simulink model "mavsim_manual_multi"  (R2016b)
settings: Solver=ode15s  StartTime=0.0  StopTime=10000  RelTol=1e-3  EnableMultiTasking=on
InitFcn:
  | param
values from neighbouring files (symbols this model uses):
  P = GenCoefs(P)    [param.m]    (also in param_chap5.m)
undefined symbols (not defined in the file or in its folder): autopilot, drawAircraft, estimate_states, forces_moments, gps, plane_follow, plotextramavstatevariables, plotmavstatevariables, sensors, true_states
libraries: simulink x9
settings Model: Creator=beard  LastModifiedBy=Brian Jackson
settings DataIOCC: LimitDataPoints=on  SaveFormat=Array  SignalLoggingSaveFormat=ModelDataLogs
settings OptimizationCC: ExpressionDepthLimit=2147483647  InitFltsAndDblsToZero=on  LifeSpan=inf
settings DebuggingCC: UnderspecifiedInitializationDetection=Classic  MergeDetectMultiDrivingBlocksExec=none  SolverPrmCheckMsg=warning  FcnCallInpInsideContextMsg=warning  StateNameClashWarn=warning  SFUnexpectedBacktrackingDiag=warning  SFNoUnconditionalDefaultTransitionDiag=warning  SFExecutionAtInitializationDiag=none
settings HardwareCC: ProdBitPerPointer=32  ProdBitPerSizeT=32  ProdBitPerPtrDiffT=32  ProdLargestAtomicFloat=None  ProdIntDivRoundTo=Undefined  ProdEndianess=Unspecified  ProdWordSize=32  ProdHWDeviceType=32-bit Generic
settings ModelReferenceCC: PropagateSignalLabelsOutOfModel=off
settings GRTTargetCC: TargetLangStandard=C89/C90 (ANSI)  GeneratePreprocessorConditionals=Disable all  CombineOutputUpdateFcns=off  GRTInterface=on
settings ConfigComp: CovMetricSettings=dw  CovHtmlReporting=on  CovSaveCumulativeToWorkspaceVar=on  CovSaveSingleToWorkspaceVar=on  CovExternalEMLEnable=off  CovSFcnEnable=off

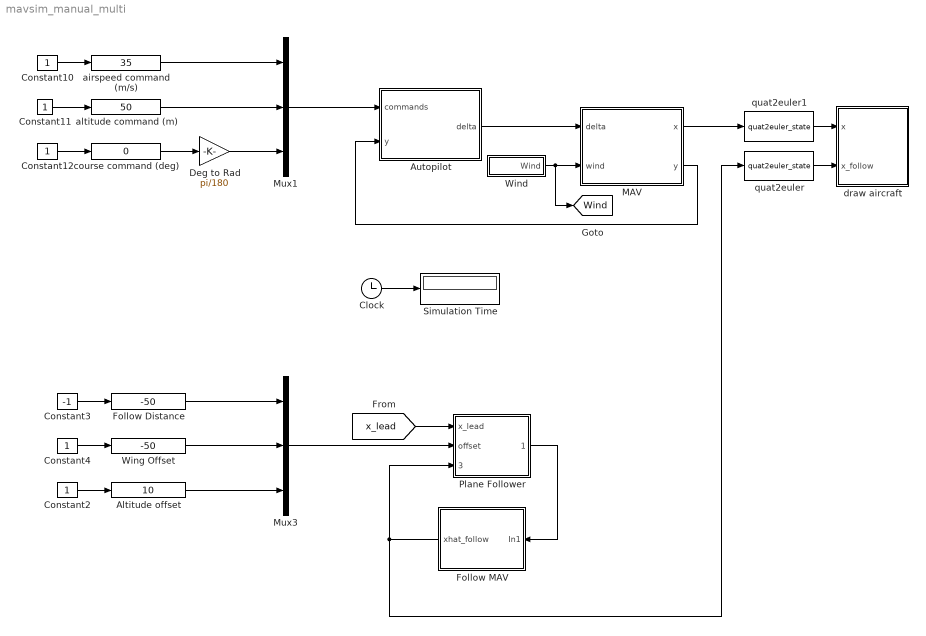
== system mavsim_manual_multi ==
  Altitude offset : simulink/Math Operations/Slider Gain  low=0  gain=10  high=10
  Autopilot : Subsystem
      mask Display: image(imread('kestrel.jpg'))
  Clock : Clock
  Constant{2,4,10..12} (5 alike) : Constant
  Constant3 : Constant  Value=-1
  Deg to Rad : Gain  Gain=pi/180
  Follow Distance : simulink/Math Operations/Slider Gain  low=-50  gain=-50  high=50
  Follow MAV : Subsystem
      mask Display: image(imread('batcam.png'))
  MAV : Subsystem
      mask Display: image(imread('batcam.png'))
  Mux1 : Mux  Inputs=3
  Mux3 : Mux  Inputs=3
  Plane Follower : Subsystem
  Simulation Time : Display
  Wind : Subsystem
  Wing Offset : simulink/Math Operations/Slider Gain  low=-50  gain=-50  high=50
  airspeed command (m/s) : simulink/Math Operations/Slider Gain  low=5  gain=35  high=50
  altitude command (m) : simulink/Math Operations/Slider Gain  low=-50  gain=50  high=500
  course command (deg) : simulink/Math Operations/Slider Gain  low=-360  gain=0  high=360
  draw aircraft : Subsystem
      mask Display: image(imread('tv.png'))
  quat2euler : MATLABFcn  MATLABFcn=quat2euler_state
  "quat2euler1 " : MATLABFcn  MATLABFcn=quat2euler_state
  tag scope: Wind=global
  wires:
  Clock/1 -> Simulation Time/1
  Autopilot/1(delta) -> MAV/1(delta)
  "quat2euler1 "/1 -> draw aircraft/1(x)
  Constant10/1 -> airspeed command (m/s)/1
  Constant11/1 -> altitude command (m)/1
  Constant12/1 -> course command (deg)/1
  course command (deg)/1 -> Deg to Rad/1
  altitude command (m)/1 -> Mux1/2
  airspeed command (m/s)/1 -> Mux1/1
  Deg to Rad/1 -> Mux1/3
  Mux1/1 -> Autopilot/1(commands)
  MAV/1(x) -> "quat2euler1 "/1
  MAV/2(y) -> Autopilot/2(y)
  Constant2/1 -> Altitude offset/1
  Constant3/1 -> Follow Distance/1
  Constant4/1 -> Wing Offset/1
  Follow Distance/1 -> Mux3/1
  Wing Offset/1 -> Mux3/2
  Altitude offset/1 -> Mux3/3
  quat2euler/1 -> draw aircraft/2(x_follow)
  Wind/1(Wind) -> [Wind], MAV/2(wind)
  [x_lead] -> Plane Follower/1(x_lead)
  Mux3/1 -> Plane Follower/2(offset)
  Follow MAV/1(xhat_follow) -> Plane Follower/3(x_follow), quat2euler/1
  Plane Follower/1(commands) -> Follow MAV/1(In1)

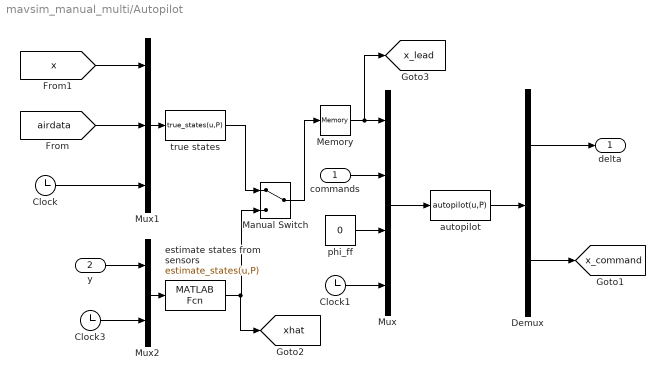
== system mavsim_manual_multi/Autopilot ==
  commands : Inport
  y : Inport  Port=2
  Clock : Clock
  Clock1 : Clock
  Clock3 : Clock
  Demux : Demux  Outputs=[4;12]
  Manual Switch : ManualSwitch
  Memory : Memory
  Mux : Mux
  Mux1 : Mux  Inputs=3
  Mux2 : Mux  Inputs=2
  autopilot : MATLABFcn  MATLABFcn=autopilot(u,P)  OutputDimensions=4+12  SampleTime=P.Ts
  estimate states from sensors : MATLABFcn  MATLABFcn=estimate_states(u,P)  OutputDimensions=19  SampleTime=P.Ts
  phi_ff : Constant  Value=0
  true states : MATLABFcn  MATLABFcn=true_states(u,P)  OutputDimensions=19  SampleTime=P.Ts
  delta : Outport
  tag scope: x_command=global, x_lead=global, xhat=global
  wires:
  Mux/1 -> autopilot/1
  Clock/1 -> Mux1/3
  autopilot/1 -> Demux/1
  Demux/1 -> delta/1
  Demux/2 -> [x_command]
  commands/1 -> Mux/2
  Mux1/1 -> true states/1
  [x] -> Mux1/1
  [airdata] -> Mux1/2
  Memory/1 -> [x_lead], Mux/1
  Clock1/1 -> Mux/4
  Mux2/1 -> estimate states from sensors/1
  y/1 -> Mux2/1
  Clock3/1 -> Mux2/2
  true states/1 -> Manual Switch/1
  estimate states from sensors/1 -> [xhat], Manual Switch/2
  Manual Switch/1 -> Memory/1
  phi_ff/1 -> Mux/3

== system mavsim_manual_multi/Follow MAV ==
  In1 : Inport
  Autopilot_follow : Subsystem
      mask Display: image(imread('kestrel.jpg'))
  MAV_follow : Subsystem
      mask Display: image(imread('batcam.png'))
  xhat_follow : Outport
  wires:
  In1/1 -> Autopilot_follow/1(commands)
  MAV_follow/1(y) -> Autopilot_follow/2(y)
  Autopilot_follow/2(delta) -> MAV_follow/1(delta)
  [Wind] -> MAV_follow/2(wind)
  Autopilot_follow/1(xhat_follow) -> xhat_follow/1

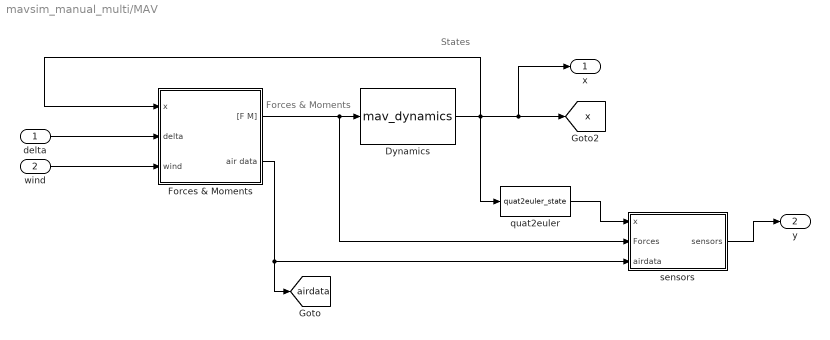
== system mavsim_manual_multi/MAV ==
  note: Forces & Moments
  note: States
  delta : Inport
  wind : Inport  Port=2
  Dynamics : S-Function  FunctionName=mav_dynamics  Parameters=P  SFunctionDeploymentMode=off  EnableBusSupport=off
  Forces & Moments : Subsystem
  "quat2euler " : MATLABFcn  MATLABFcn=quat2euler_state
  sensors : Subsystem
  x : Outport
  y : Outport  Port=2
  tag scope: airdata=global, x=global
  wires:
  Dynamics/1 -> x/1, [x], Forces & Moments/1(x), "quat2euler "/1
  Forces & Moments/1("[F M]") -> sensors/2(Forces), Dynamics/1
  Forces & Moments/2(air data) -> sensors/3(airdata), [airdata]
  delta/1 -> Forces & Moments/2(delta)
  wind/1 -> Forces & Moments/3(wind)
  "quat2euler "/1 -> sensors/1(x)
  sensors/1(sensors) -> y/1

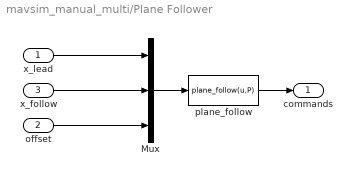
== system mavsim_manual_multi/Plane Follower ==
  x_lead : Inport
  offset : Inport  Port=2
  x_follow : Inport  Port=3
  Mux : Mux  Inputs=3
  plane_follow : MATLABFcn  MATLABFcn=plane_follow(u,P)  OutputDimensions=4
  commands : Outport
  wires:
  offset/1 -> Mux/3
  Mux/1 -> plane_follow/1
  x_lead/1 -> Mux/1
  x_follow/1 -> Mux/2
  plane_follow/1 -> commands/1

== system mavsim_manual_multi/Wind ==
  Constant1 : Constant  Value=[0; 0; 0]
  Constant2 : Constant  Value=[P.wind_n; P.wind_e; P.wind_d]
  Mux1 : Mux  Inputs=2
  Wind Gusts : Subsystem
  Wind : Outport
  wires:
  Constant2/1 -> Mux1/1
  Mux1/1 -> Wind/1
  Constant1/1 -> Mux1/2

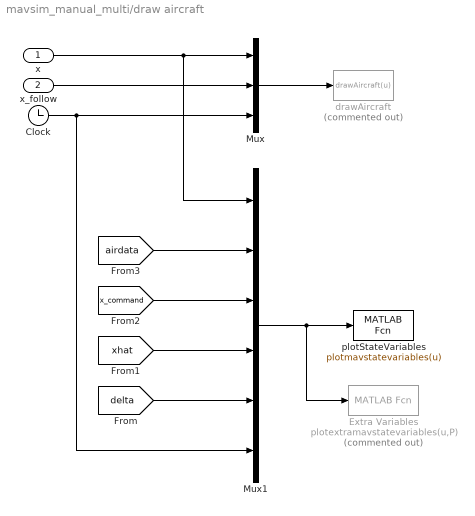
== system mavsim_manual_multi/draw aircraft ==
  x : Inport
  x_follow : Inport  Port=2
  Clock : Clock
  Extra Variables : MATLABFcn  Commented=on  MATLABFcn=plotextramavstatevariables(u,P)  OutputDimensions=0
  Mux : Mux  Inputs=3
  Mux1 : Mux  Inputs=6
  drawAircraft : MATLABFcn  Commented=on  MATLABFcn=drawAircraft(u)  OutputDimensions=0  SampleTime=0.1
  plotStateVariables : MATLABFcn  MATLABFcn=plotmavstatevariables(u)  OutputDimensions=0  SampleTime=0.1
  wires:
  Mux/1 -> drawAircraft/1
  x/1 -> Mux1/1, Mux/1
  Clock/1 -> Mux/3, Mux1/6
  Mux1/1 -> Extra Variables/1, plotStateVariables/1
  [xhat] -> Mux1/4
  [x_command] -> Mux1/3
  [delta] -> Mux1/5
  [airdata] -> Mux1/2
  x_follow/1 -> Mux/2

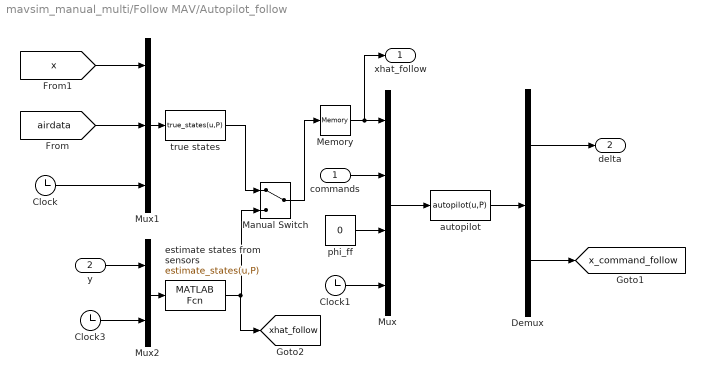
== system mavsim_manual_multi/Follow MAV/Autopilot_follow ==
  commands : Inport
  y : Inport  Port=2
  Clock : Clock
  Clock1 : Clock
  Clock3 : Clock
  Demux : Demux  Outputs=[4;12]
  Manual Switch : ManualSwitch
  Memory : Memory
  Mux : Mux
  Mux1 : Mux  Inputs=3
  Mux2 : Mux  Inputs=2
  autopilot : MATLABFcn  MATLABFcn=autopilot(u,P)  OutputDimensions=4+12  SampleTime=P.Ts
  estimate states from sensors : MATLABFcn  MATLABFcn=estimate_states(u,P)  OutputDimensions=19  SampleTime=P.Ts
  phi_ff : Constant  Value=0
  true states : MATLABFcn  MATLABFcn=true_states(u,P)  OutputDimensions=19  SampleTime=P.Ts
  xhat_follow : Outport
  delta : Outport  Port=2
  tag scope: x_command_follow=global, xhat_follow=global
  wires:
  Mux/1 -> autopilot/1
  Clock/1 -> Mux1/3
  autopilot/1 -> Demux/1
  Demux/1 -> delta/1
  Demux/2 -> [x_command_follow]
  commands/1 -> Mux/2
  Mux1/1 -> true states/1
  [x] -> Mux1/1
  [airdata] -> Mux1/2
  Memory/1 -> xhat_follow/1, Mux/1
  Clock1/1 -> Mux/4
  Mux2/1 -> estimate states from sensors/1
  y/1 -> Mux2/1
  Clock3/1 -> Mux2/2
  true states/1 -> Manual Switch/1
  estimate states from sensors/1 -> [xhat_follow], Manual Switch/2
  Manual Switch/1 -> Memory/1
  phi_ff/1 -> Mux/3

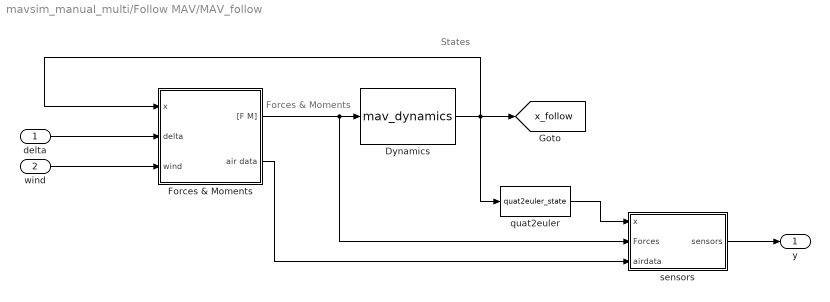
== system mavsim_manual_multi/Follow MAV/MAV_follow ==
  note: Forces & Moments
  note: States
  delta : Inport
  wind : Inport  Port=2
  Dynamics : S-Function  FunctionName=mav_dynamics  Parameters=P  SFunctionDeploymentMode=off  EnableBusSupport=off
  Forces & Moments : Subsystem
  "quat2euler " : MATLABFcn  MATLABFcn=quat2euler_state
  sensors : Subsystem
  y : Outport
  tag scope: x_follow=global
  wires:
  Dynamics/1 -> [x_follow], Forces & Moments/1(x), "quat2euler "/1
  Forces & Moments/1("[F M]") -> sensors/2(Forces), Dynamics/1
  Forces & Moments/2(air data) -> sensors/3(airdata)
  delta/1 -> Forces & Moments/2(delta)
  wind/1 -> Forces & Moments/3(wind)
  "quat2euler "/1 -> sensors/1(x)
  sensors/1(sensors) -> y/1

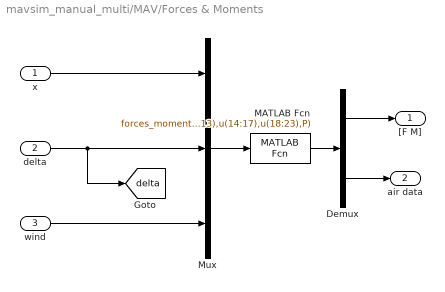
== system mavsim_manual_multi/MAV/Forces & Moments ==
  x : Inport
  delta : Inport  Port=2
  wind : Inport  Port=3
  Demux : Demux  Outputs=[6;6]
  MATLAB Fcn : MATLABFcn  MATLABFcn=forces_moments(u(1:13),u(14:17),u(18:23),P)  OutputDimensions=12
  Mux : Mux  Inputs=3
  "[F M]" : Outport
  air data : Outport  Port=2
  tag scope: delta=global
  wires:
  Demux/2 -> air data/1
  Mux/1 -> MATLAB Fcn/1
  Demux/1 -> "[F M]"/1
  MATLAB Fcn/1 -> Demux/1
  wind/1 -> Mux/3
  delta/1 -> Mux/2, [delta]
  x/1 -> Mux/1

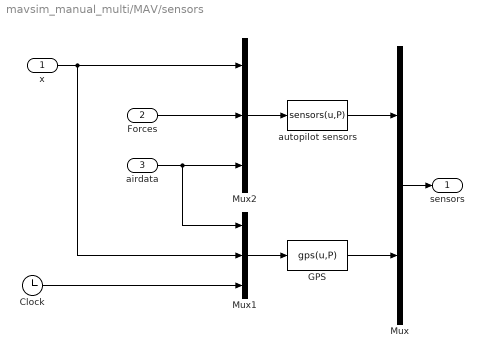
== system mavsim_manual_multi/MAV/sensors ==
  x : Inport
  Forces : Inport  Port=2
  airdata : Inport  Port=3
  Clock : Clock
  GPS : MATLABFcn  MATLABFcn=gps(u,P)  OutputDimensions=5  SampleTime=P.Ts_gps
  Mux : Mux  Inputs=2
  Mux1 : Mux  Inputs=3
  Mux2 : Mux  Inputs=3
  autopilot sensors : MATLABFcn  MATLABFcn=sensors(u,P)  OutputDimensions=8  SampleTime=P.Ts
  sensors : Outport
  wires:
  autopilot sensors/1 -> Mux/1
  GPS/1 -> Mux/2
  Mux1/1 -> GPS/1
  Clock/1 -> Mux1/3
  Mux2/1 -> autopilot sensors/1
  Forces/1 -> Mux2/2
  airdata/1 -> Mux2/3, Mux1/1
  Mux/1 -> sensors/1
  x/1 -> Mux2/1, Mux1/2

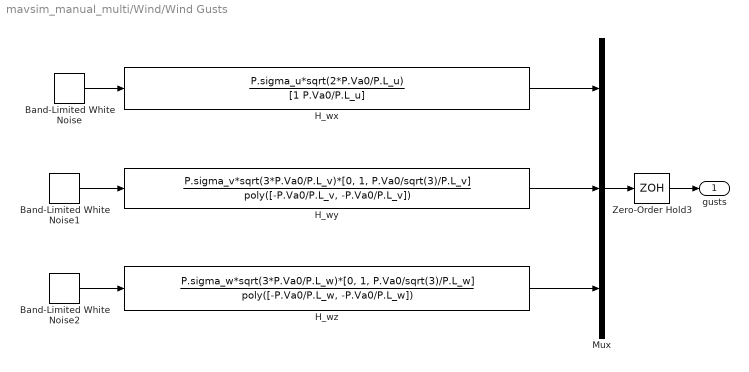
== system mavsim_manual_multi/Wind/Wind Gusts ==
  Band-Limited White Noise : simulink/Sources/Band-Limited White Noise  Cov=[1]  Ts=P.Ts  seed=[23341]
  Band-Limited White Noise1 : simulink/Sources/Band-Limited White Noise  Cov=[1]  Ts=P.Ts  seed=[23341]
  Band-Limited White Noise2 : simulink/Sources/Band-Limited White Noise  Cov=[1]  Ts=P.Ts  seed=[23341]
  H_wx : TransferFcn  Numerator=P.sigma_u*sqrt(2*P.Va0/P.L_u)  Denominator=[1 P.Va0/P.L_u]
  H_wy : TransferFcn  Numerator=P.sigma_v*sqrt(3*P.Va0/P.L_v)*[0, 1, P.Va0/sqrt(3)/P.L_v]  Denominator=poly([-P.Va0/P.L_v, -P.Va0/P.L_v])
  H_wz : TransferFcn  Numerator=P.sigma_w*sqrt(3*P.Va0/P.L_w)*[0, 1, P.Va0/sqrt(3)/P.L_w]  Denominator=poly([-P.Va0/P.L_w, -P.Va0/P.L_w])
  Mux : Mux  Inputs=3
  Zero-Order Hold3 : ZeroOrderHold  SampleTime=P.Ts
  gusts : Outport
  wires:
  H_wx/1 -> Mux/1
  Band-Limited White Noise/1 -> H_wx/1
  H_wy/1 -> Mux/2
  Band-Limited White Noise1/1 -> H_wy/1
  H_wz/1 -> Mux/3
  Band-Limited White Noise2/1 -> H_wz/1
  Mux/1 -> Zero-Order Hold3/1
  Zero-Order Hold3/1 -> gusts/1

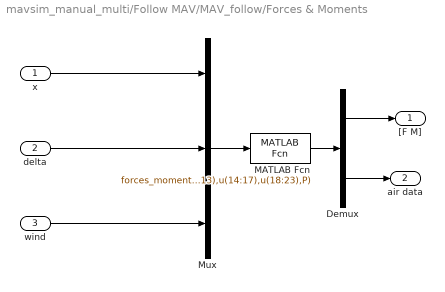
== system mavsim_manual_multi/Follow MAV/MAV_follow/Forces & Moments ==
  x : Inport
  delta : Inport  Port=2
  wind : Inport  Port=3
  Demux : Demux  Outputs=[6;6]
  MATLAB Fcn : MATLABFcn  MATLABFcn=forces_moments(u(1:13),u(14:17),u(18:23),P)  OutputDimensions=12
  Mux : Mux  Inputs=3
  "[F M]" : Outport
  air data : Outport  Port=2
  wires:
  Demux/2 -> air data/1
  Mux/1 -> MATLAB Fcn/1
  Demux/1 -> "[F M]"/1
  MATLAB Fcn/1 -> Demux/1
  wind/1 -> Mux/3
  delta/1 -> Mux/2
  x/1 -> Mux/1

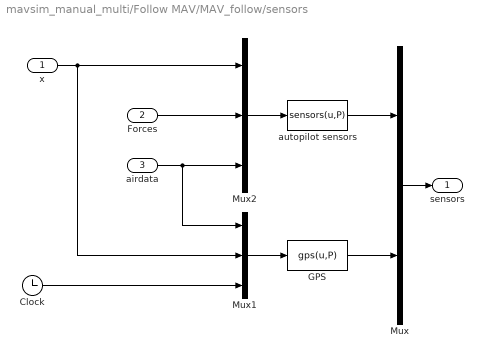
== system mavsim_manual_multi/Follow MAV/MAV_follow/sensors ==
  x : Inport
  Forces : Inport  Port=2
  airdata : Inport  Port=3
  Clock : Clock
  GPS : MATLABFcn  MATLABFcn=gps(u,P)  OutputDimensions=5  SampleTime=P.Ts_gps
  Mux : Mux  Inputs=2
  Mux1 : Mux  Inputs=3
  Mux2 : Mux  Inputs=3
  autopilot sensors : MATLABFcn  MATLABFcn=sensors(u,P)  OutputDimensions=8  SampleTime=P.Ts
  sensors : Outport
  wires:
  autopilot sensors/1 -> Mux/1
  GPS/1 -> Mux/2
  Mux1/1 -> GPS/1
  Clock/1 -> Mux1/3
  Mux2/1 -> autopilot sensors/1
  Forces/1 -> Mux2/2
  airdata/1 -> Mux2/3, Mux1/1
  Mux/1 -> sensors/1
  x/1 -> Mux2/1, Mux1/2
